simulink model "hydra_leg"  (R2014b)
settings: configuration reference "HardwareConfig" (kept outside this file)
undefined symbols (not defined in the file or in its folder): gcbh, LCD_Status, NXTFcns, rmidispblock, Speak
libraries: legoev3lib x6, ControllersFcns x2, simulink x1
PreSaveFcn:
  | % Creates new data dictionary based on template.
  | 
  | projRoot = ETRoboconUtilities.getCheckoutRoot;
  | dictName = [bdroot 'Data.sldd'];
  | 
  | source = fullfile(projRoot,'templates','RobotTemplateData.sldd');
  | dest = fullfile(projRoot,'data_dictionaries',dictName);
  | 
  | if ~exist(dest) && ~isequal(bdroot,'RobotTemplate')
  |   copyfile(source,dest);
  |   disp(['Created new dictionary ' dictName ' in the data_dictionaries folder.']);
  |   set_param(bdroot,'DataDictionary', dictName);
  | end
Description:
  | ET Robocon 2014 robot template model.
  | 
  | Author:  Sebastian Castro
settings Model: DataDictionary=hydra_legData.sldd  ExtModeTrigDuration=2  Creator=mbiesiad  LastModifiedBy=pkaniara

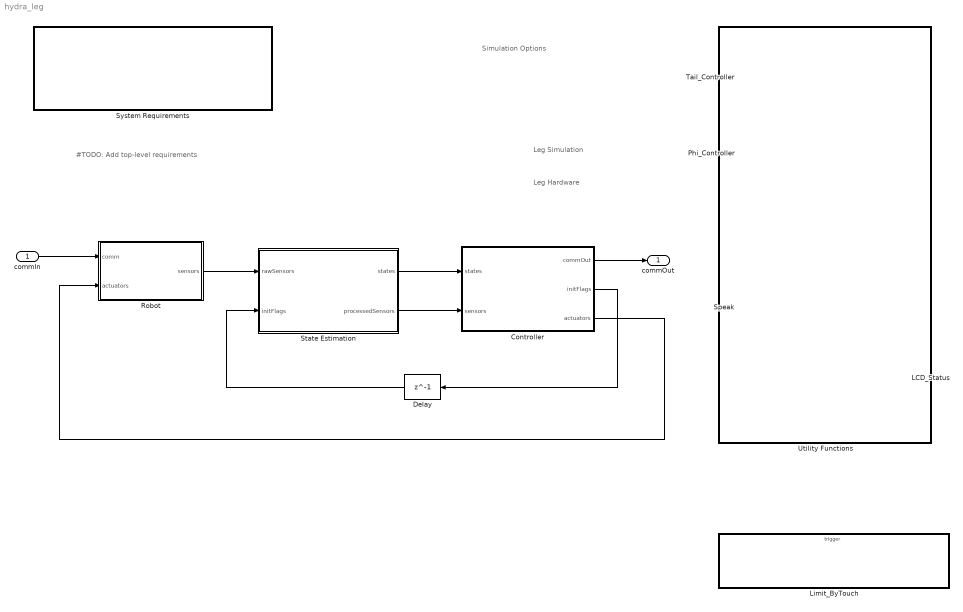
== system hydra_leg ==
  note: #TODO:
      | Add top-level requirements
  note: Simulation Options
  note: Leg Hardware
  note: Leg Simulation
  commIn : Inport
  Controller : Stateflow chart  TreatAsAtomicUnit=on
  Delay : Delay  DelayLength=1
      settings: AttributesFormatString=Removes algebraic loop
  LCD_Status : Subsystem  AncestorBlock=NXTFcns/LCD_Status  TreatAsAtomicUnit=on
  Limit_ByTouch : Subsystem  TreatAsAtomicUnit=on
  Phi_Controller : ControllersFcns/Phi_Controller
  Robot : Subsystem  Variant=on  VariantControl=Variant1
  Speak : Subsystem  AncestorBlock=NXTFcns/Speak  TreatAsAtomicUnit=on
  State Estimation : Subsystem
  System Requirements : Subsystem  LoadFcn=rmidispblock('load',gcbh)  mask(System Requirements){id=SystemReq, title=System Requirements}
      mask prompts: title "Block Title"
      mask help: Lists the requirements for the current model.
      mask init:
      | id = 'SystemReq';
      | [w,h] = rmidispblock('display',gcbh);
      settings: CopyFcn=rmidispblock('create',gcbh)  DeleteFcn=rmidispblock('delete',gcbh)  ModelCloseFcn=rmidispblock('close',gcbh)  PreSaveFcn=rmidispblock('close',gcbh)  PostSaveFcn=rmidispblock('open',gcbh)  OpenFcn=rmidispblock('open',gcbh)  MoveFcn=rmidispblock('move',gcbh)
      mask Help: helpview(fullfile(docroot,'toolbox','slvnv','slvnv.map'),'systemrequirements')
      mask Display:
      | text(326/2,113-4,rmidispblock('title',gcbh),'horizontalAlignment','center','verticalAlignment','top')
      | text(w/2,h/2,'<No Requirements in System>','horizontalAlignment','center','verticalAlignment','top')
  Tail_Controller : ControllersFcns/Tail_Controller
  Utility Functions : Subsystem
  commOut : Outport
  wires:
  State Estimation/2(processedSensors) -> Controller/2(sensors)
  Robot/1(sensors) -> State Estimation/1(rawSensors)
  Controller/2(initFlags) -> Delay/1
  State Estimation/1(states) -> Controller/1(states)
  Delay/1 -> State Estimation/2(initFlags)
  Controller/3(actuators) -> Robot/2(actuators)
  Controller/1(commOut) -> commOut/1
  commIn/1 -> Robot/1(comm)

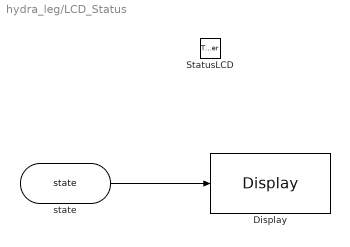
== system hydra_leg/LCD_Status ==
  StatusLCD : TriggerPort  TriggerType=function-call  IsSimulinkFunction=on  FunctionName=StatusLCD
  Display : legoev3lib/Display  slcdLine=1  slcdFormat=Decimal
  state : ArgIn  OutDataTypeStr=uint16  ArgumentName=state
  wires:
  state/1 -> Display/1

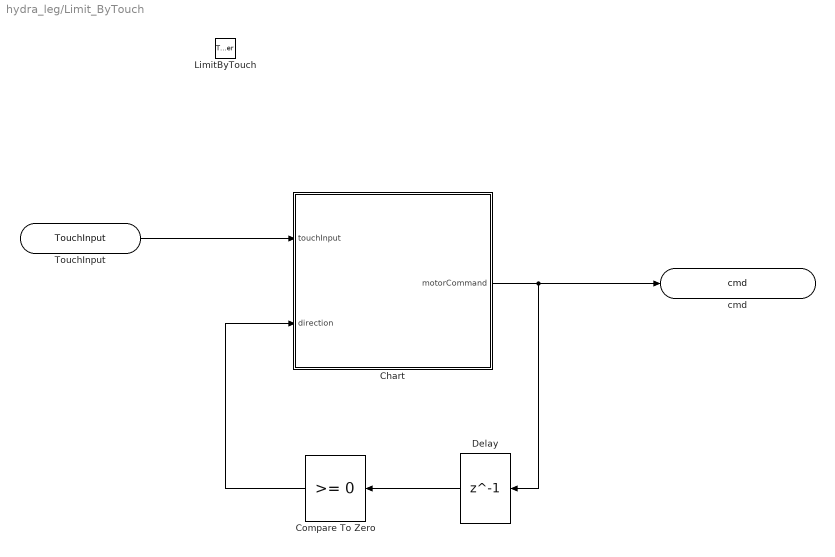
== system hydra_leg/Limit_ByTouch ==
  LimitByTouch : TriggerPort  TriggerType=function-call  IsSimulinkFunction=on  FunctionName=LimitByTouch
  Chart : Stateflow chart  TreatAsAtomicUnit=on
  Compare To Zero : simulink/Logic and Bit Operations/Compare To Zero  relop=>=  OutDataTypeStr=boolean
  Delay : Delay  DelayLength=1
  TouchInput : ArgIn  DisableCoverage=on  ArgumentName=TouchInput
  cmd : ArgOut  DisableCoverage=on  ArgumentName=cmd
  wires:
  TouchInput/1 -> Chart/1(touchInput)
  Chart/1(motorCommand) -> Delay/1, cmd/1
  Delay/1 -> Compare To Zero/1
  Compare To Zero/1 -> Chart/2(direction)

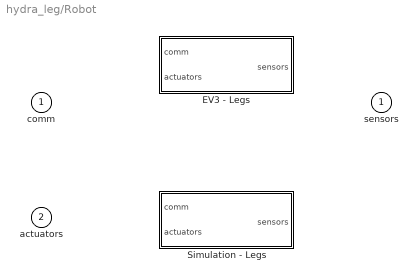
== system hydra_leg/Robot ==
  comm : Inport
  actuators : Inport  Port=2
  EV3 - Legs : Subsystem  VariantControl=HardwareVar
  Simulation - Legs : Subsystem  VariantControl=SimulationVar
  sensors : Outport

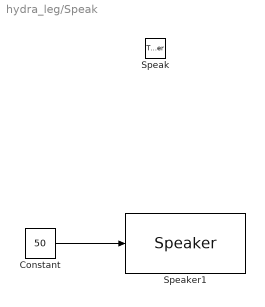
== system hydra_leg/Speak ==
  Speak : TriggerPort  TriggerType=function-call  IsSimulinkFunction=on  FunctionName=Speak
  Constant : Constant  Value=50
  Speaker1 : legoev3lib/Speaker  sinputMode=Volume only  sspeakerFreq=100  sspeakerVolume=50  sspeakerDuration=100
  wires:
  Constant/1 -> Speaker1/1

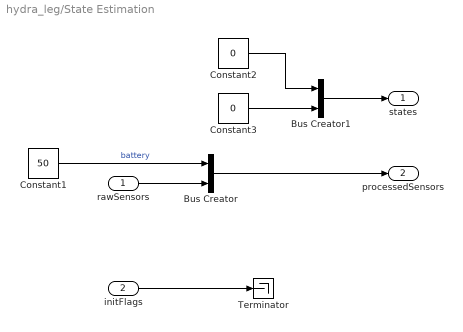
== system hydra_leg/State Estimation ==
  rawSensors : Inport
  initFlags : Inport  Port=2  OutDataTypeStr=Bus: Init_Bus
  Bus Creator : BusCreator  Inputs='battery','touch'  OutDataTypeStr=Bus: Sensors_Bus
  Bus Creator1 : BusCreator  Inputs=2  OutDataTypeStr=Bus: States_Bus
      settings: InheritFromInputs=off
  Constant1 : Constant  Value=50
  Constant2 : Constant  Value=0
  Constant3 : Constant  Value=0
  Terminator : Terminator
  states : Outport
  processedSensors : Outport  Port=2
  wires:
  Bus Creator1/1 -> states/1
  initFlags/1 -> Terminator/1
  Bus Creator/1 -> processedSensors/1
  Constant1/1 -> Bus Creator/1  "battery"
  rawSensors/1 -> Bus Creator/2
  Constant3/1 -> Bus Creator1/2
  Constant2/1 -> Bus Creator1/1

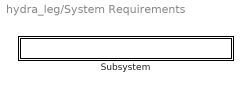
== system hydra_leg/System Requirements ==
  Subsystem : Subsystem  mask{label=0, index=1}
      mask init:
      | label = rmidispblock('label',index);
      settings: OpenFcn=rmidispblock('openReq',gcbh);
      mask Display: text(0,0,label,'horizontalAlignment','left','verticalAlignment','bottom')

== system hydra_leg/Utility Functions ==

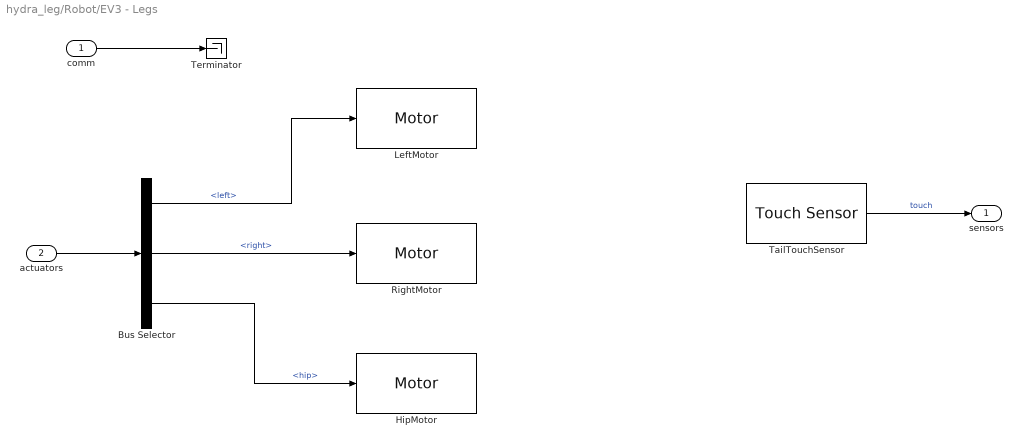
== system hydra_leg/Robot/EV3 - Legs ==
  comm : Inport
  actuators : Inport  Port=2
  Bus Selector : BusSelector  OutputSignals=left,right,hip
  HipMotor : legoev3lib/Motor  sportNumber=C  sstopAction=Brake
  LeftMotor : legoev3lib/Motor  sportNumber=A  sstopAction=Brake
  RightMotor : legoev3lib/Motor  sportNumber=B  sstopAction=Brake
  TailTouchSensor : legoev3lib/Touch Sensor  portNumber=1  sampleTime=0.1
  Terminator : Terminator
  sensors : Outport
  wires:
  comm/1 -> Terminator/1
  TailTouchSensor/1 -> sensors/1  "touch"
  Bus Selector/1 -> LeftMotor/1  "<left>"
  actuators/1 -> Bus Selector/1
  Bus Selector/2 -> RightMotor/1  "<right>"
  Bus Selector/3 -> HipMotor/1  "<hip>"

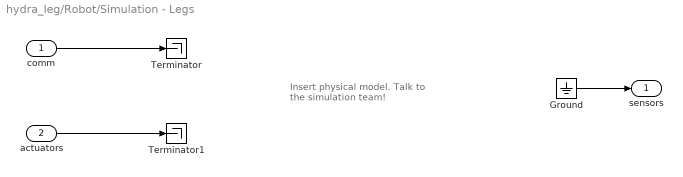
== system hydra_leg/Robot/Simulation - Legs ==
  note: Insert physical model.
      | Talk to the simulation team!
  comm : Inport
  actuators : Inport  Port=2
  Ground : Ground
  Terminator : Terminator
  Terminator1 : Terminator
  sensors : Outport
  wires:
  comm/1 -> Terminator/1
  actuators/1 -> Terminator1/1
  Ground/1 -> sensors/1

== system hydra_leg/System Requirements/Subsystem ==

== stateflow chart hydra_leg/Limit_ByTouch/Chart ==
  state Clockwise
    en,du:
    motorCommand = 20;
  state AntiClockwise
    en,du:
    motorCommand = -20;
  AntiClockwise -> Clockwise : [direction==0 && touchInput ==1]
  Clockwise -> AntiClockwise : [direction==1 && touchInput ==1]
  data: touchInput input; motorCommand output; direction input

== stateflow chart hydra_leg/Controller ==
  note: #TODO
      | Add requirements to Stateflow objects
      | by right-clicking and selecting the
      | Requirements Traceability option.
  state LegAction
    entry:
    %initializing
    actuators.right = single(0);
    actuators.left = single(0);
    actuators.hip = single(0);
    initFlags.tail = single(0);
    initFlags.fall = single(0);
    du:
    commOut = single(0);
    state Stationary
    state StraightForward
    state CurvePath
    (default) -> Stationary
    Stationary -> StraightForward : after(5,sec)
    StraightForward -> CurvePath : after (10,sec)
  (default) -> LegAction
  data: commOut output single size=1; states input Bus: States_Bus size=1; sensors input Bus: Sensors_Bus size=1; initFlags output Bus: Init_Bus size=1; actuators output Bus: Actuators_bus size=1
